simulink model "original"  (R2015a)
settings: Solver=ode45  StartTime=0.0  StopTime=2000  RelTol=1e-3
values from neighbouring files (symbols this model uses):
  alpha = a(i)    [AsymOscillPeriods.m]    (also in averagedRelayOutput.m = alphaArray(i); bursting_linearised.m = 0.5; compareApproximations.m = 0.5; evaluateDerivatives.m = variables(3))
  alpha_const = 0.0    (= 0)    [averagedRelayOutput.m]    (also in bursting_linearised.m = 0.1; fastSlow.m; manParamsNullclines.m; manipulateParameters.m = getappdata(hObject.Parent,'alpha_const'))
  alpha_delay1 = 4000    [fast_nullcline_winged_cusp.m]    (also in ode_slider_demo.m = 200; originalModel.m = 300; originalModel2.m = 300; piece_wise_model.m = 200)
  alpha_delay2 = 7000    [fast_nullcline_winged_cusp.m]    (also in ode_slider_demo.m = 300; originalModel.m = 200; originalModel2.m = 200; piece_wise_model.m = 300)
  alpha_max = 1    [fast_nullcline_winged_cusp.m]    (also in ode_slider_demo.m = 1.75; originalModel.m = 0.5; originalModel2.m = 0.5; piece_wise_model.m = 1.75)
  alpha_period = t_max    (= 10000)    [fast_nullcline_winged_cusp.m]    (also in ode_slider_demo.m = 3500; originalModel.m = 1400; originalModel2.m = 6000; piece_wise_model.m)
  alpha_width = 1    [fast_nullcline_winged_cusp.m]    (also in ode_slider_demo.m; originalModel.m = 0.1; originalModel2.m = 0.1; piece_wise_model.m)
  beta = 0.37    [averagedRelayOutput.m]    (also in bursting_linearised.m = 0.27; compareApproximations.m = 1.5; fastSlow.m; fast_nullcline_winged_cusp.m = 0.5)
  delta = 0.5    [averagedRelayOutput.m]    (also in bursting_linearised.m; compareApproximations.m; fastSlow.m; fast_nullcline_winged_cusp.m)
  fast_plant_X0 = -1.0    (= -1)    [averagedRelayOutput.m]    (also in bursting_linearised.m = -1.05; fastSlow.m; fast_nullcline_winged_cusp.m; hRose.m = 0)
  gamma = 0    [averagedRelayOutput.m]    (also in bursting_linearised.m = 1; compareApproximations.m = 1; fastSlow.m; fast_nullcline_winged_cusp.m = 1)
  slow_plant_X0 = -1.0    (= -1)    [averagedRelayOutput.m]    (also in bursting_linearised.m = -1.05; fastSlow.m; fast_nullcline_winged_cusp.m = -2; hRose.m = -10)
  ts = 1    [averagedRelayOutput.m]    (also in bursting_linearised.m; compareApproximations.m; fastSlow.m; fast_nullcline_winged_cusp.m)
  tus = 800    [averagedRelayOutput.m]    (also in bursting_linearised.m; fastSlow.m; manParamsNullclines.m; manipulateParameters.m = getappdata(hObject.Parent,'tus'))
  ultra_slow_plant_X0 = 0.45    [averagedRelayOutput.m]    (also in bursting_linearised.m = 0; fastSlow.m; hRose.m = 2000; manParamsNullclines.m)
settings Model: Creator=ra428  LastModifiedBy=ra428

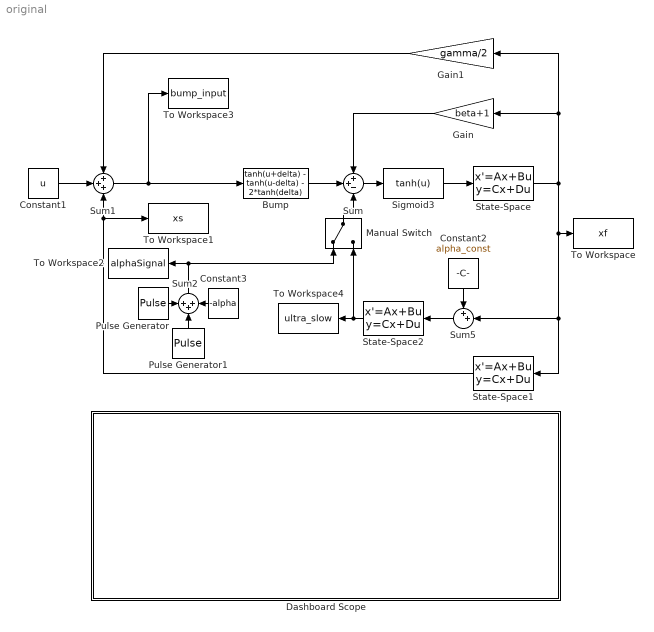
== system original ==
  Bump : Fcn  Expr="tanh(u+delta) -  tanh(u-delta) - 2*tanh(delta)"
  Constant1 : Constant  Value=u
  Constant2 : Constant  Value=alpha_const
  Constant3 : Constant  Value=-alpha
  Dashboard Scope : Subsystem  DialogController=hmiCreateDDGDialog  IsWebBlock=on  mask(MathWorksWebBlock){webBlockId=eea715ed-5406-42a9-88e4-354f31446561, webBlockType=sdiscope, ShowInitialText=on, HMISrcModelName=original}
      mask prompts: webBlockId "WebBlock Id"; webBlockType "WebBlock Type"; HMISrcModelName "Source Model"
      mask Help: helpview([docroot '/mapfiles/simulink.map'], 'hmi_scope')
      mask Display:
      | if strcmp(get_param(bdroot(gcb),'BlockDiagramType'), 'library')
      |     image([(matlabroot) '/toolbox/simulink/hmi/icons/DashboardScope.png']);
      | end
  Gain : Gain  Gain=beta+1
  Gain1 : Gain  Gain=gamma/2
  Manual Switch : ManualSwitch
  Pulse Generator : DiscretePulseGenerator  PulseType=Time based  Amplitude=alpha_max  Period=alpha_period  PulseWidth=alpha_width  PhaseDelay=alpha_delay1
  Pulse Generator1 : DiscretePulseGenerator  PulseType=Time based  Amplitude=-1*alpha_max  Period=alpha_period  PulseWidth=alpha_width  PhaseDelay=alpha_delay2
  Sigmoid3 : Fcn  Expr=tanh(u)
  State-Space : StateSpace  A=-1/tf  B=1/tf  D=0  X0=fast_plant_X0
  State-Space1 : StateSpace  A=-1/ts  B=1/ts  D=0  X0=slow_plant_X0
  State-Space2 : StateSpace  A=-1/tus  B=1/tus  D=0  X0=ultra_slow_plant_X0
  Sum : Sum  Inputs=++-
  Sum1 : Sum  Inputs=+++
  Sum2 : Sum  Inputs=+++
  Sum5 : Sum  Inputs=++|
  To Workspace : ToWorkspace  VariableName=xf  SaveFormat=Timeseries  SampleTime=-1
  To Workspace1 : ToWorkspace  VariableName=xs  SaveFormat=Timeseries  SampleTime=-1
  To Workspace2 : ToWorkspace  VariableName=alphaSignal  SaveFormat=Timeseries  SampleTime=-1
  To Workspace3 : ToWorkspace  VariableName=bump_input  SaveFormat=Timeseries  SampleTime=-1
  To Workspace4 : ToWorkspace  VariableName=ultra_slow  SaveFormat=Timeseries  SampleTime=-1
  wires:
  Sum/1 -> Sigmoid3/1
  Sum1/1 -> Bump/1, To Workspace3/1
  Gain/1 -> Sum/1
  Gain1/1 -> Sum1/1
  Sigmoid3/1 -> State-Space/1
  State-Space/1 -> State-Space1/1, Sum5/2, To Workspace/1, Gain/1, Gain1/1
  State-Space1/1 -> Sum1/3, To Workspace1/1
  Constant2/1 -> Sum5/1
  Sum5/1 -> State-Space2/1
  State-Space2/1 -> Manual Switch/2, To Workspace4/1
  Bump/1 -> Sum/2
  Constant1/1 -> Sum1/2
  Pulse Generator1/1 -> Sum2/2
  Manual Switch/1 -> Sum/3
  Pulse Generator/1 -> Sum2/1
  Constant3/1 -> Sum2/3
  Sum2/1 -> Manual Switch/1, To Workspace2/1

== system original/Dashboard Scope ==
